simulink model "questao4_simulink"  (R2022b)
settings: Solver=VariableStepAuto  StartTime=0.0  StopTime=0.1  RelTol=1e-3
model workspace (MAT data in the model file):
  C = 0.0008
  L = 0.001
  R = 1
  Vi = 1
settings Model: Creator=pedro  LastModifiedBy=maria

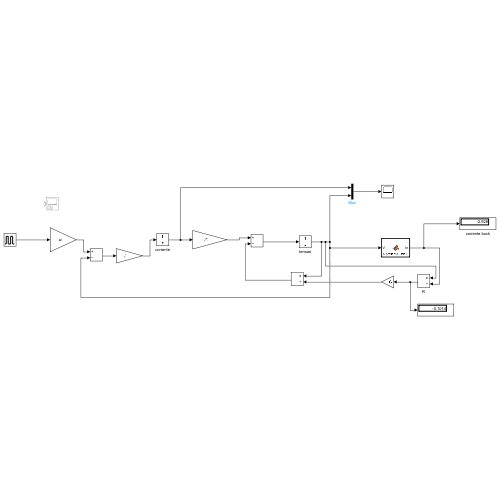
[thumbnail: Simulink's stored preview of the top-level diagram]
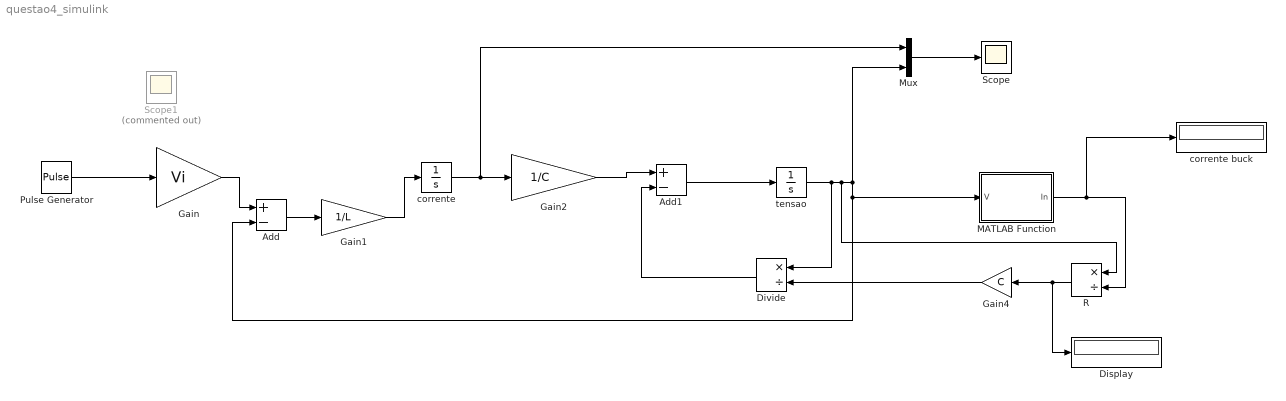
== system questao4_simulink ==
  Add : Sum  Inputs=+-
  Add1 : Sum  Inputs=+-
  Display : Display
  Divide : Product  Inputs=*/  RndMeth=Zero  SaturateOnIntegerOverflow=on
  Gain : Gain  Gain=Vi
  Gain1 : Gain  Gain=1/L
  Gain2 : Gain  Gain=1/C
  Gain4 : Gain  Gain=C
  MATLAB Function : MATLAB Function  TreatAsAtomicUnit=on
  Mux : Mux  Inputs=2
  Pulse Generator : DiscretePulseGenerator  PulseType=Time based  Period=1/(2*10^3)  PulseWidth=30
  R : Product  Inputs=*/  RndMeth=Zero  SaturateOnIntegerOverflow=on
  Scope : Scope
  Scope1 : Scope  Commented=on
  corrente : Integrator
  corrente buck : Display
  tensao : Integrator  InitialCondition=1
  wires:
  corrente/1 -> Mux/1, Gain2/1
  Mux/1 -> Scope/1
  Gain/1 -> Add/1
  Add1/1 -> tensao/1
  Gain2/1 -> Add1/1
  Add/1 -> Gain1/1
  Gain1/1 -> corrente/1
  Pulse Generator/1 -> Gain/1
  Gain4/1 -> Divide/2
  tensao/1 -> Divide/1, R/1, MATLAB Function/1(V), Add/2, Mux/2
  MATLAB Function/1(In) -> corrente buck/1, R/2
  R/1 -> Display/1, Gain4/1
  Divide/1 -> Add1/2

== matlab function questao4_simulink/MATLAB Function ==
  data: V input; In output
function In = resistencia_celula(V)

Gn = 1000; %[W/m^2] irradiação solar nominal
G = Gn; %[W/m^2] irradiação solar
Isen = 3.1656; %[A] corrente de curto-circuito nominal
Ki = 1.8*10^-3; %[A/◦C] coef. de temperatura da corrente de curto-circuito
Tn = 298; %[K] temp. nominal da célula fotovoltaica
Rp = 38.17; %[Ω] resistência paralela (shunt)
A = 1.7538; %fator de idealidade do diodo
Rs = 61.3*10^-3; %[Ω] resistência série
Is = 5.68*10^-6; %[A] corrente de saturação do diodo (valor nominal) 



k = 1.38*10^-23; %[J/K] constante de Boltzmann
q = 1.602*10^-19; %[C] carga do elétron
T = 298; %[K] temperatura da célula

Vt = (k*T)/q;
tol = 0.001;
lambda = 0.3;
In = 0;



var = 10*tol;
iter = 0;
while (abs(var) > tol && iter <= 1000)

    Ia = In;
    
    Ipv = (G/Gn)*(Isen+Ki*(T-Tn));
   
    Id = Is*(exp((V+Rs*Ia)/(Vt*A))-1);
  
    Ip = (V+(Rs*Ia))/Rp;
    
    In = Ipv - Id - Ip;
    In = lambda*In + (1-lambda)*Ia; %corrente da célula
    
    var = In-Ia;
    iter = iter +1;
    
end

In = -In; %corrente do buck
return
